simulink model "CLSC_BLDCM_with_Hallsensor"  (R2014b)
settings: Solver=ode3  StartTime=0.0  StopTime=0.2  FixedStep=1e-5  MaxStep=1e-5  RelTol=1e-3
settings Model: Creator=Rhoever  LastModifiedBy=root

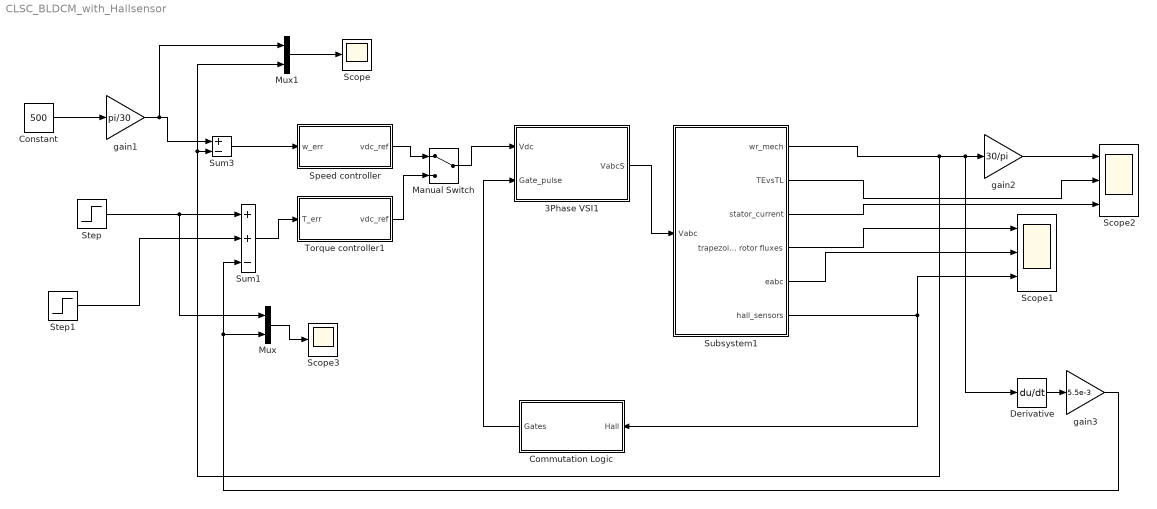
== system CLSC_BLDCM_with_Hallsensor ==
  3Phase VSI1 : Subsystem
  Commutation Logic : Subsystem
  Constant : Constant  Value=500
  Derivative : Derivative
  Manual Switch : ManualSwitch
  Mux : Mux  Inputs=2
  Mux1 : Mux  Inputs=2
  Scope : Scope
      settings: SaveName=ScopeData3
  Scope1 : Scope  NumInputPorts=3
      settings: YMin=-75~-110~-0.2  YMax=75~110~1.2
  Scope2 : Scope  NumInputPorts=3
      settings: YMin=-75~-3~-15  YMax=75~2.5~20
  Scope3 : Scope
      settings: YMin=0  YMax=1  SaveName=ScopeData2
  Speed controller : Subsystem
  Step : Step  Time=0.5  After=2  SampleTime=0
  Step1 : Step  After=-1  SampleTime=0
  Subsystem1 : Subsystem  mask(BLDC Motor :){Rs=1.43, Lls=9.4e-3, Phi_m=0.2158, J=5.5e-3, B=2e-3, P=4}
      mask prompts: Rs "Resistance - Rs [ohms]"; Lls "Inductance - Lls [H]"; Phi_m "Rotor Flux [wb]"; J "Rotor Inertia - J [kg-m^2]"; B "Friction Coefficient -B"; P "No of Poles"
      mask init:
      | Trap=0.5;
      mask Display: fprintf('BLDC Motor')
  Sum1 : Sum  Inputs=++-
  Sum3 : Sum  Inputs=+-
  Torque controller1 : Subsystem
  gain1 : Gain  Gain=pi/30  SaturateOnIntegerOverflow=on  OutDataTypeStr=Inherit: Same as input  ParamDataTypeStr=Inherit: Same as input
  gain2 : Gain  Gain=30/pi  SaturateOnIntegerOverflow=on  OutDataTypeStr=Inherit: Same as input  ParamDataTypeStr=Inherit: Same as input
  gain3 : Gain  Gain=5.5e-3  SaturateOnIntegerOverflow=on  OutDataTypeStr=Inherit: Same as input  ParamDataTypeStr=Inherit: Same as input
  wires:
  Subsystem1/6(hall_sensors) -> Scope1/3, Commutation Logic/1("Hall ")
  Subsystem1/4(trapezoidal rotor fluxes) -> Scope1/1
  Subsystem1/3(stator_current) -> Scope2/3
  Subsystem1/2(TEvsTL) -> Scope2/2
  Subsystem1/5(eabc) -> Scope1/2
  3Phase VSI1/1(VabcS) -> Subsystem1/1(Vabc)
  Commutation Logic/1(Gates) -> 3Phase VSI1/2(Gate_pulse)
  Sum3/1 -> Speed controller/1(w_err)
  Manual Switch/1 -> 3Phase VSI1/1(Vdc)
  Subsystem1/1(wr_mech) -> Derivative/1, gain2/1, Mux1/2, Sum3/2
  gain2/1 -> Scope2/1
  Constant/1 -> gain1/1
  gain1/1 -> Mux1/1, Sum3/1
  Derivative/1 -> gain3/1
  gain3/1 -> Sum1/3, Mux/2
  Sum1/1 -> Torque controller1/1(T_err)
  Speed controller/1(vdc_ref) -> Manual Switch/1
  Torque controller1/1(vdc_ref) -> Manual Switch/2
  Mux/1 -> Scope3/1
  Step/1 -> Mux/1, Sum1/1
  Step1/1 -> Sum1/2
  Mux1/1 -> Scope/1

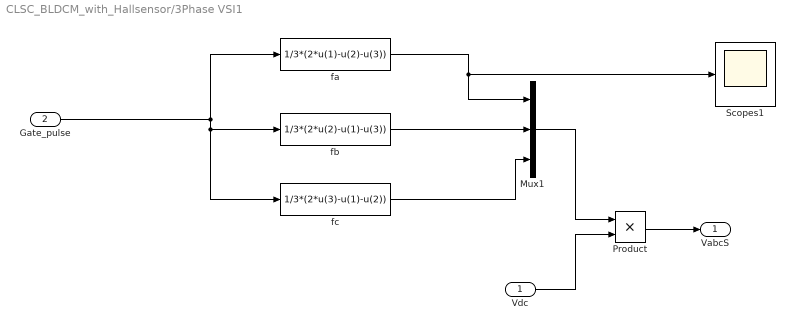
== system CLSC_BLDCM_with_Hallsensor/3Phase VSI1 ==
  Vdc : Inport
  Gate_pulse : Inport  Port=2
  Mux1 : Mux  Inputs=3
  Product : Product
  Scopes1 : Scope
      settings: TimeRange=0.04  YMin=-40  YMax=40  SaveName=ScopeData5
  fa : Fcn  Expr=1/3*(2*u(1)-u(2)-u(3))
  fb : Fcn  Expr=1/3*(2*u(2)-u(1)-u(3))
  fc : Fcn  Expr=1/3*(2*u(3)-u(1)-u(2))
  VabcS : Outport
  wires:
  Gate_pulse/1 -> fa/1, fb/1, fc/1
  fb/1 -> Mux1/2
  fc/1 -> Mux1/3
  fa/1 -> Scopes1/1, Mux1/1
  Mux1/1 -> Product/1
  Product/1 -> VabcS/1
  Vdc/1 -> Product/2

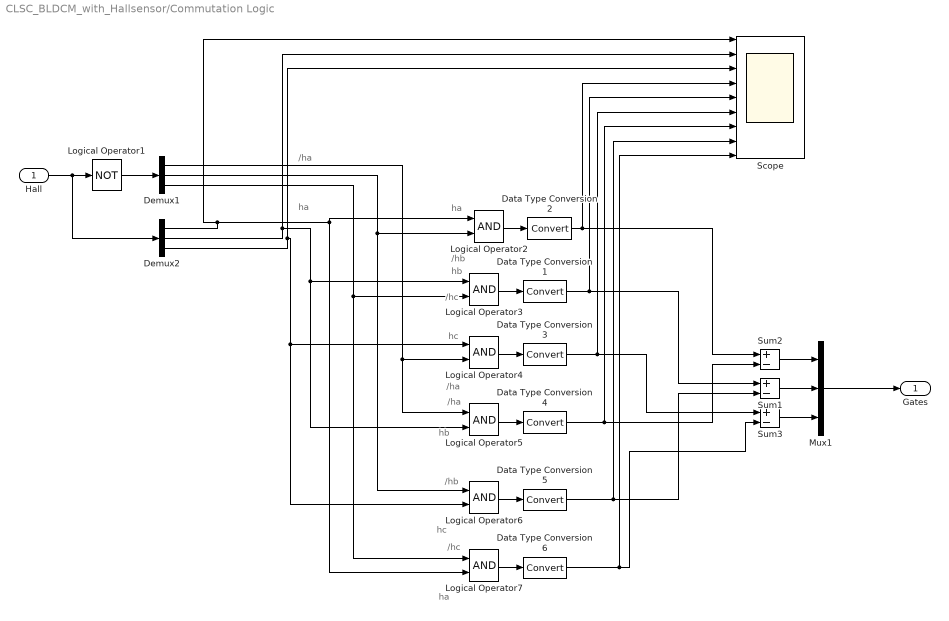
== system CLSC_BLDCM_with_Hallsensor/Commutation Logic ==
  note: ha
  note: /hc
  note: hc
  note: /hb
  note: hb
  note: /ha
  note: /ha
  note: hc
  note: /hc
  note: hb
  note: /hb
  note: ha
  note: ha
  note: /ha
  "Hall " : Inport
  Data Type Conversion{1..6} (6 alike) : DataTypeConversion
  Demux1 : Demux  Outputs=3
  Demux2 : Demux  Outputs=3
  Logical Operator1 : Logic  Operator=NOT  AllPortsSameDT=off  OutDataTypeStr=boolean
  Logical Operator{2..7} (6 alike) : Logic  AllPortsSameDT=off  OutDataTypeStr=boolean
  Mux1 : Mux  Inputs=3
  Scope : Scope  NumInputPorts=9
      settings: YMin=0~0~0~0~0~0~0~0~0  YMax=1~1~1~1~1~1~1~1~1  SaveName=ScopeData4
  Sum1 : Sum  Inputs=+-  OutDataTypeStr=double
  Sum2 : Sum  Inputs=+-  OutDataTypeStr=double
  Sum3 : Sum  Inputs=+-  OutDataTypeStr=double
  Gates : Outport
  wires:
  Demux2/3 -> Scope/3, Logical Operator6/2, Logical Operator4/1
  Sum2/1 -> Mux1/1
  Mux1/1 -> Gates/1
  Logical Operator1/1 -> Demux1/1
  Logical Operator7/1 -> Data Type Conversion6/1
  Sum3/1 -> Mux1/3
  Logical Operator4/1 -> Data Type Conversion3/1
  Data Type Conversion4/1 -> Scope/7, Sum2/2
  Data Type Conversion5/1 -> Scope/8, Sum1/2
  Demux1/1 -> Logical Operator5/1, Logical Operator4/2
  Data Type Conversion3/1 -> Scope/6, Sum3/1
  Data Type Conversion6/1 -> Scope/9, Sum3/2
  Logical Operator5/1 -> Data Type Conversion4/1
  Data Type Conversion2/1 -> Scope/4, Sum2/1
  Logical Operator6/1 -> Data Type Conversion5/1
  Demux1/2 -> Logical Operator6/1, Logical Operator2/2
  Logical Operator2/1 -> Data Type Conversion2/1
  Logical Operator3/1 -> Data Type Conversion1/1
  "Hall "/1 -> Demux2/1, Logical Operator1/1
  Data Type Conversion1/1 -> Scope/5, Sum1/1
  Sum1/1 -> Mux1/2
  Demux2/2 -> Scope/2, Logical Operator5/2, Logical Operator3/1
  Demux1/3 -> Logical Operator7/1, Logical Operator3/2
  Demux2/1 -> Scope/1, Logical Operator2/1, Logical Operator7/2

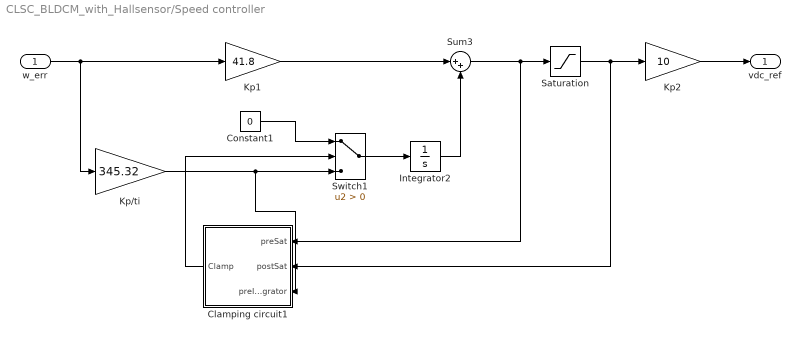
== system CLSC_BLDCM_with_Hallsensor/Speed controller ==
  w_err : Inport
  Clamping circuit1 : Subsystem
  Constant1 : Constant  DisableCoverage=on  Value=0  OutDataTypeStr=Inherit: Inherit via back propagation  PreserveConstantTs=on
  Integrator2 : Integrator
  Kp/ti : Gain  Gain=345.32
  Kp1 : Gain  Gain=41.8
  Kp2 : Gain  Gain=10
  Saturation : Saturate  UpperLimit=15  LowerLimit=-15
  Sum3 : Sum  Inputs=|++
  Switch1 : Switch  DisableCoverage=on  Criteria=u2 > Threshold  InputSameDT=on
  vdc_ref : Outport
  wires:
  Kp1/1 -> Sum3/1
  Sum3/1 -> Saturation/1, Clamping circuit1/1(preSat)
  Saturation/1 -> Kp2/1, Clamping circuit1/2(postSat)
  w_err/1 -> Kp/ti/1, Kp1/1
  Kp2/1 -> vdc_ref/1
  Integrator2/1 -> Sum3/2
  Kp/ti/1 -> Switch1/3, Clamping circuit1/3(preIntegrator)
  Clamping circuit1/1(Clamp) -> Switch1/2
  Switch1/1 -> Integrator2/1
  Constant1/1 -> Switch1/1

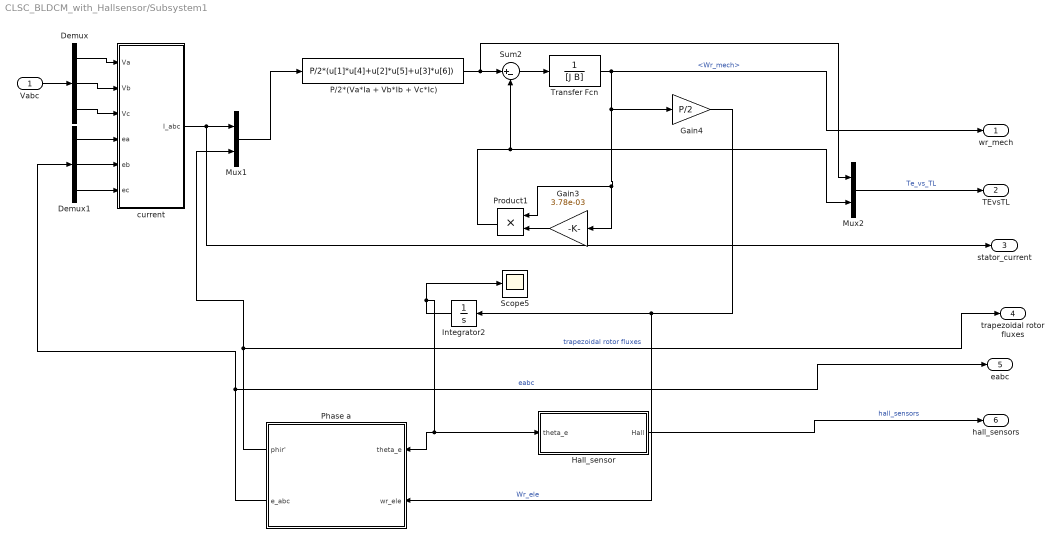
== system CLSC_BLDCM_with_Hallsensor/Subsystem1 ==
  Vabc : Inport
  Demux : Demux  Outputs=3
  Demux1 : Demux  Outputs=3
  Gain3 : Gain  Gain=3.78e-03
  Gain4 : Gain  Gain=P/2
  Hall_sensor : Subsystem
  Integrator2 : Integrator
  Mux1 : Mux  Inputs=2
  Mux2 : Mux  Inputs=2
  P/2*(Va*Ia + Vb*Ib + Vc*Ic) : Fcn  Expr=P/2*(u[1]*u[4]+u[2]*u[5]+u[3]*u[6])
  Phase a : Subsystem
  Product1 : Product
  Scope5 : Scope
      settings: TimeRange=2  YMin=22.7  YMax=24.1  SaveName=ScopeData6
  Sum2 : Sum  Inputs=|+-
  Transfer Fcn : TransferFcn  Denominator=[J B]
  current : Subsystem
  wr_mech : Outport
  TEvsTL : Outport  Port=2
  stator_current : Outport  Port=3
  trapezoidal rotor fluxes : Outport  Port=4
  eabc : Outport  Port=5
  hall_sensors : Outport  Port=6
  wires:
  Demux/3 -> current/3(Vc)
  Demux/1 -> current/1(Va)
  Demux/2 -> current/2(Vb)
  Sum2/1 -> Transfer Fcn/1
  Vabc/1 -> Demux/1
  Mux1/1 -> P/2*(Va*Ia + Vb*Ib + Vc*Ic)/1
  Demux1/3 -> current/6(ec)
  Demux1/2 -> current/5(eb)
  Demux1/1 -> current/4(ea)
  Integrator2/1 -> Phase a/1(theta_e), Hall_sensor/1(theta_e), Scope5/1
  Product1/1 -> Sum2/2, Mux2/2
  Phase a/2(e_abc) -> eabc/1, Demux1/1  "eabc"
  Gain4/1 -> Phase a/2(wr_ele), Integrator2/1  "Wr_ele"
  Phase a/1(phir') -> trapezoidal rotor fluxes/1, Mux1/2  "trapezoidal rotor fluxes"
  current/1(I_abc) -> stator_current/1, Mux1/1
  P/2*(Va*Ia + Vb*Ib + Vc*Ic)/1 -> Mux2/1, Sum2/1
  Hall_sensor/1(Hall) -> hall_sensors/1  "hall_sensors"
  Mux2/1 -> TEvsTL/1  "Te_vs_TL"
  Transfer Fcn/1 -> wr_mech/1, Gain3/1, Product1/1, Gain4/1  "<Wr_mech>"
  Gain3/1 -> Product1/2

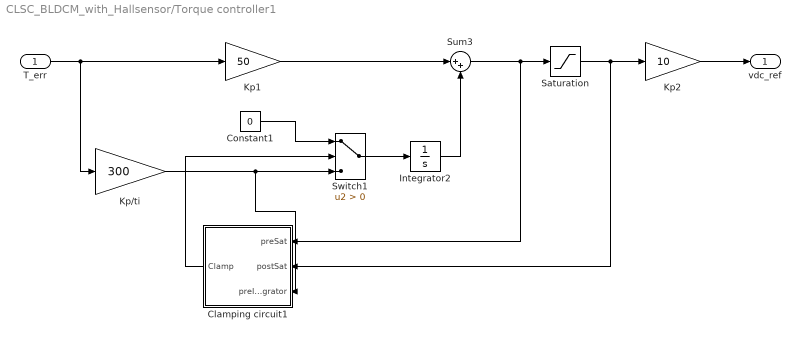
== system CLSC_BLDCM_with_Hallsensor/Torque controller1 ==
  T_err : Inport
  Clamping circuit1 : Subsystem
  Constant1 : Constant  DisableCoverage=on  Value=0  OutDataTypeStr=Inherit: Inherit via back propagation  PreserveConstantTs=on
  Integrator2 : Integrator
  Kp/ti : Gain  Gain=300
  Kp1 : Gain  Gain=50
  Kp2 : Gain  Gain=10
  Saturation : Saturate  UpperLimit=15  LowerLimit=-15
  Sum3 : Sum  Inputs=|++
  Switch1 : Switch  DisableCoverage=on  Criteria=u2 > Threshold  InputSameDT=on
  vdc_ref : Outport
  wires:
  Kp1/1 -> Sum3/1
  Sum3/1 -> Saturation/1, Clamping circuit1/1(preSat)
  Saturation/1 -> Kp2/1, Clamping circuit1/2(postSat)
  T_err/1 -> Kp/ti/1, Kp1/1
  Kp2/1 -> vdc_ref/1
  Integrator2/1 -> Sum3/2
  Kp/ti/1 -> Switch1/3, Clamping circuit1/3(preIntegrator)
  Clamping circuit1/1(Clamp) -> Switch1/2
  Switch1/1 -> Integrator2/1
  Constant1/1 -> Switch1/1

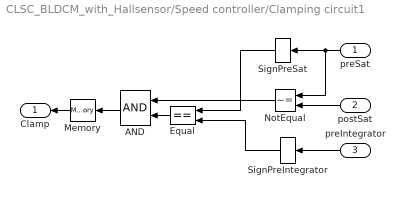
== system CLSC_BLDCM_with_Hallsensor/Speed controller/Clamping circuit1 ==
  preSat : Inport
  postSat : Inport  Port=2
  preIntegrator : Inport  Port=3
  AND : Logic  DisableCoverage=on  OutDataTypeStr=boolean
  Equal : RelationalOperator  DisableCoverage=on  Operator===  OutDataTypeStr=boolean  InputSameDT=on
  Memory : Memory
  NotEqual : RelationalOperator  DisableCoverage=on  Operator=~=  OutDataTypeStr=boolean  InputSameDT=on
  SignPreIntegrator : Signum  DisableCoverage=on
  SignPreSat : Signum  DisableCoverage=on
  Clamp : Outport
  wires:
  Memory/1 -> Clamp/1
  AND/1 -> Memory/1
  Equal/1 -> AND/2
  SignPreIntegrator/1 -> Equal/2
  NotEqual/1 -> AND/1
  SignPreSat/1 -> Equal/1
  preIntegrator/1 -> SignPreIntegrator/1
  postSat/1 -> NotEqual/2
  preSat/1 -> NotEqual/1, SignPreSat/1

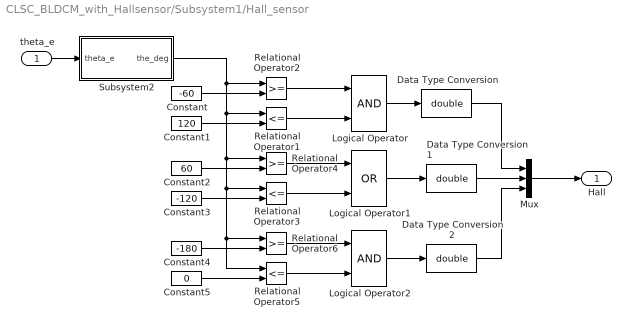
== system CLSC_BLDCM_with_Hallsensor/Subsystem1/Hall_sensor ==
  theta_e : Inport
  Constant : Constant  Value=-60
  Constant1 : Constant  Value=120
  Constant2 : Constant  Value=60
  Constant3 : Constant  Value=-120
  Constant4 : Constant  Value=-180
  Constant5 : Constant  Value=0
  Data Type Conversion : DataTypeConversion  OutDataTypeStr=double  SaturateOnIntegerOverflow=on  RndMeth=Zero
  Data Type Conversion1 : DataTypeConversion  OutDataTypeStr=double  SaturateOnIntegerOverflow=on  RndMeth=Zero
  Data Type Conversion2 : DataTypeConversion  OutDataTypeStr=double  SaturateOnIntegerOverflow=on  RndMeth=Zero
  Logical Operator : Logic  AllPortsSameDT=off  OutDataTypeStr=boolean
  Logical Operator1 : Logic  Operator=OR  AllPortsSameDT=off  OutDataTypeStr=boolean
  Logical Operator2 : Logic  AllPortsSameDT=off  OutDataTypeStr=boolean
  Mux : Mux  Inputs=3
  Relational Operator1 : RelationalOperator  Operator=<=  InputSameDT=on
  Relational Operator2 : RelationalOperator  InputSameDT=on
  Relational Operator3 : RelationalOperator  Operator=<=  InputSameDT=on
  Relational Operator4 : RelationalOperator  InputSameDT=on
  Relational Operator5 : RelationalOperator  Operator=<=  InputSameDT=on
  Relational Operator6 : RelationalOperator  InputSameDT=on
  Subsystem2 : Subsystem
  Hall : Outport
  wires:
  Constant3/1 -> Relational Operator3/2
  Data Type Conversion2/1 -> Mux/3
  Data Type Conversion1/1 -> Mux/2
  Data Type Conversion/1 -> Mux/1
  Relational Operator5/1 -> Logical Operator2/2
  Logical Operator2/1 -> Data Type Conversion2/1
  Relational Operator6/1 -> Logical Operator2/1
  Constant4/1 -> Relational Operator6/2
  Constant5/1 -> Relational Operator5/2
  Relational Operator3/1 -> Logical Operator1/2
  Logical Operator1/1 -> Data Type Conversion1/1
  Logical Operator/1 -> Data Type Conversion/1
  Mux/1 -> Hall/1
  Relational Operator2/1 -> Logical Operator/1
  Relational Operator1/1 -> Logical Operator/2
  Subsystem2/1(the_deg) -> Relational Operator4/1, Relational Operator3/1, Relational Operator5/1, Relational Operator6/1, Relational Operator1/1, Relational Operator2/1
  Constant/1 -> Relational Operator2/2
  Relational Operator4/1 -> Logical Operator1/1
  Constant1/1 -> Relational Operator1/2
  Constant2/1 -> Relational Operator4/2
  theta_e/1 -> Subsystem2/1(theta_e)

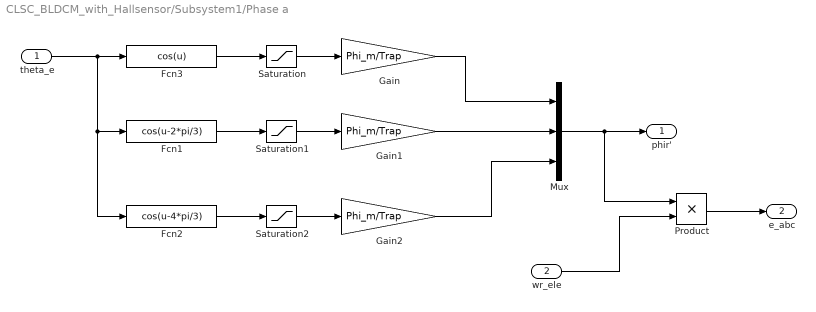
== system CLSC_BLDCM_with_Hallsensor/Subsystem1/Phase a ==
  theta_e : Inport
  wr_ele : Inport  Port=2
  Fcn1 : Fcn  Expr=cos(u-2*pi/3)
  Fcn2 : Fcn  Expr=cos(u-4*pi/3)
  Fcn3 : Fcn  Expr=cos(u)
  Gain : Gain  Gain=Phi_m/Trap
  Gain1 : Gain  Gain=Phi_m/Trap
  Gain2 : Gain  Gain=Phi_m/Trap
  Mux : Mux  Inputs=3
  Product : Product
  Saturation : Saturate  UpperLimit=Trap  LowerLimit=-Trap
  Saturation1 : Saturate  UpperLimit=Trap  LowerLimit=-Trap
  Saturation2 : Saturate  UpperLimit=Trap  LowerLimit=-Trap
  phir' : Outport
  e_abc : Outport  Port=2
  wires:
  Fcn3/1 -> Saturation/1
  theta_e/1 -> Fcn2/1, Fcn1/1, Fcn3/1
  Fcn2/1 -> Saturation2/1
  Fcn1/1 -> Saturation1/1
  Gain/1 -> Mux/1
  Gain1/1 -> Mux/2
  Gain2/1 -> Mux/3
  Mux/1 -> phir'/1, Product/1
  wr_ele/1 -> Product/2
  Product/1 -> e_abc/1
  Saturation/1 -> Gain/1
  Saturation1/1 -> Gain1/1
  Saturation2/1 -> Gain2/1

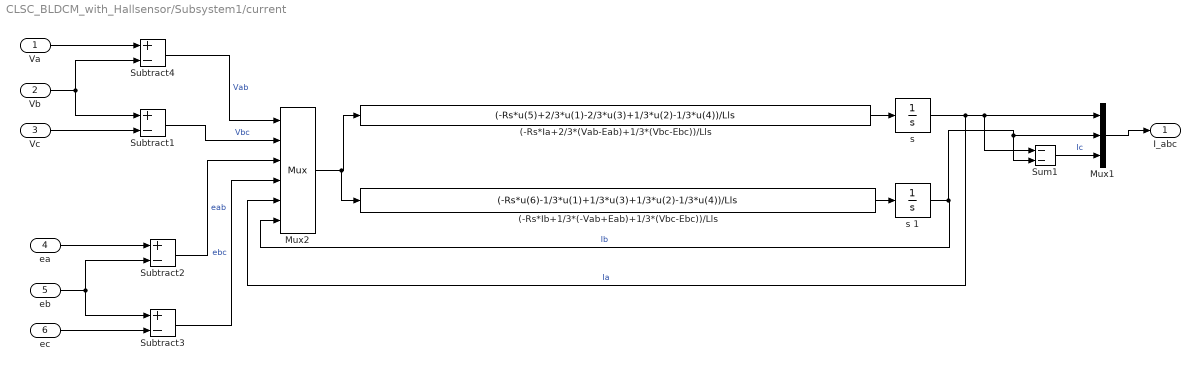
== system CLSC_BLDCM_with_Hallsensor/Subsystem1/current ==
  Va : Inport
  Vb : Inport  Port=2
  Vc : Inport  Port=3
  ea : Inport  Port=4
  eb : Inport  Port=5
  ec : Inport  Port=6
  (-Rs*Ia+2/3*(Vab-Eab)+1/3*(Vbc-Ebc))/Lls : Fcn  Expr=(-Rs*u(5)+2/3*u(1)-2/3*u(3)+1/3*u(2)-1/3*u(4))/Lls
  (-Rs*Ib+1/3*(-Vab+Eab)+1/3*(Vbc-Ebc))/Lls : Fcn  Expr=(-Rs*u(6)-1/3*u(1)+1/3*u(3)+1/3*u(2)-1/3*u(4))/Lls
  Mux1 : Mux  Inputs=3
  Mux2 : Mux  Inputs=6
      settings: DisplayOption=signals
  Subtract{1..4} (4 alike) : Sum  Inputs=+-
  Sum1 : Sum  Inputs=--  SaturateOnIntegerOverflow=on
  "s " : Integrator
  s 1 : Integrator
  I_abc : Outport
  wires:
  Va/1 -> Subtract4/1
  Vb/1 -> Subtract4/2, Subtract1/1
  Vc/1 -> Subtract1/2
  eb/1 -> Subtract2/2, Subtract3/1
  ea/1 -> Subtract2/1
  ec/1 -> Subtract3/2
  (-Rs*Ia+2/3*(Vab-Eab)+1/3*(Vbc-Ebc))/Lls/1 -> "s "/1
  Subtract3/1 -> Mux2/4  "ebc"
  (-Rs*Ib+1/3*(-Vab+Eab)+1/3*(Vbc-Ebc))/Lls/1 -> s 1/1
  Subtract4/1 -> Mux2/1  "Vab"
  Subtract1/1 -> Mux2/2  "Vbc"
  Subtract2/1 -> Mux2/3  "eab"
  Mux2/1 -> (-Rs*Ib+1/3*(-Vab+Eab)+1/3*(Vbc-Ebc))/Lls/1, (-Rs*Ia+2/3*(Vab-Eab)+1/3*(Vbc-Ebc))/Lls/1
  s 1/1 -> Sum1/2, Mux1/2, Mux2/6  "Ib"
  "s "/1 -> Sum1/1, Mux1/1, Mux2/5  "Ia"
  Sum1/1 -> Mux1/3  "Ic"
  Mux1/1 -> I_abc/1

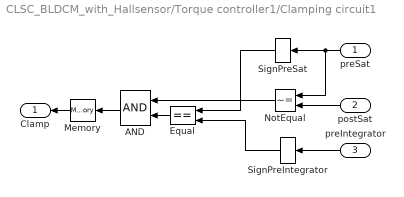
== system CLSC_BLDCM_with_Hallsensor/Torque controller1/Clamping circuit1 ==
  preSat : Inport
  postSat : Inport  Port=2
  preIntegrator : Inport  Port=3
  AND : Logic  DisableCoverage=on  OutDataTypeStr=boolean
  Equal : RelationalOperator  DisableCoverage=on  Operator===  OutDataTypeStr=boolean  InputSameDT=on
  Memory : Memory
  NotEqual : RelationalOperator  DisableCoverage=on  Operator=~=  OutDataTypeStr=boolean  InputSameDT=on
  SignPreIntegrator : Signum  DisableCoverage=on
  SignPreSat : Signum  DisableCoverage=on
  Clamp : Outport
  wires:
  Memory/1 -> Clamp/1
  AND/1 -> Memory/1
  Equal/1 -> AND/2
  SignPreIntegrator/1 -> Equal/2
  NotEqual/1 -> AND/1
  SignPreSat/1 -> Equal/1
  preIntegrator/1 -> SignPreIntegrator/1
  postSat/1 -> NotEqual/2
  preSat/1 -> NotEqual/1, SignPreSat/1

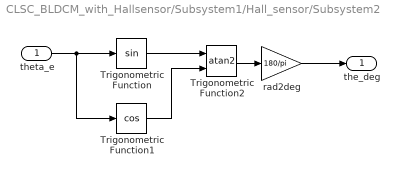
== system CLSC_BLDCM_with_Hallsensor/Subsystem1/Hall_sensor/Subsystem2 ==
  theta_e : Inport
  Trigonometric Function : Trigonometry
  Trigonometric Function1 : Trigonometry  Operator=cos
  Trigonometric Function2 : Trigonometry  Operator=atan2
  rad2deg : Gain  Gain=180/pi  SaturateOnIntegerOverflow=on  OutDataTypeStr=Inherit: Same as input  ParamDataTypeStr=Inherit: Same as input
  the_deg : Outport
  wires:
  Trigonometric Function2/1 -> rad2deg/1
  Trigonometric Function/1 -> Trigonometric Function2/1
  Trigonometric Function1/1 -> Trigonometric Function2/2
  theta_e/1 -> Trigonometric Function1/1, Trigonometric Function/1
  rad2deg/1 -> the_deg/1
